simulink model "MSD_MODEL"  (R2016a)
settings: Solver=VariableStepAuto  StartTime=0.0  StopTime=10.0  RelTol=1e-3
settings Model: Creator=Hamid  LastModifiedBy=Hamid

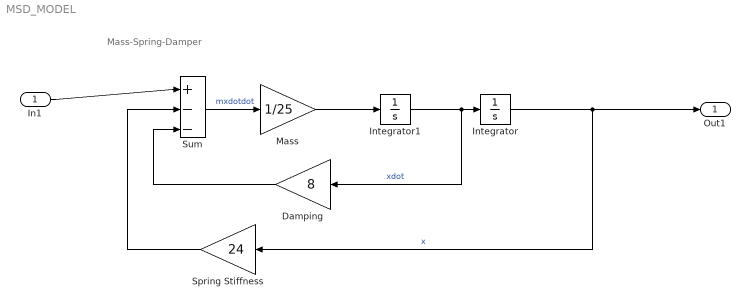
== system MSD_MODEL ==
  note: Mass-Spring-Damper
  In1 : Inport
  Damping : Gain  Gain=8
  Integrator : Integrator
  Integrator1 : Integrator
  Mass : Gain  Gain=1/25
  Spring Stiffness : Gain  Gain=24
  Sum : Sum  Inputs=|+--
  Out1 : Outport
  wires:
  Integrator/1 -> Out1/1, Spring Stiffness/1  "x"
  Integrator1/1 -> Integrator/1, Damping/1  "xdot"
  Damping/1 -> Sum/3
  Spring Stiffness/1 -> Sum/2
  Sum/1 -> Mass/1  "mxdotdot"
  Mass/1 -> Integrator1/1
  In1/1 -> Sum/1
